simulink model "MCU_vectorControl_dsPIC33AK128MC106_MCLV_48V_300W_2022a"  (R2022a)
settings: Solver=FixedStepDiscrete  StartTime=0.0  StopTime=10.0  FixedStep=50e-6  RelTol=1e-3  EnableMultiTasking=on
undefined symbols (not defined in the file or in its folder): A0, A4, ADC, B0, Bias1, Bias2, C10, C11, C6, C7, C8, control, D11, D12, DiscIntNeverNeededParam, inverter, Max, MaxPer, model, ms, NumBits1, NumBits2, P1, P17, P20, P39, P40, P41, P43, P44, P60, P61, Pin, PosRange1, PosRange2, PWM1_Trg1, Resol, s, Slope1, Slope2, us
libraries: simulink x43, MCHP_Blockset x23
(part 3 of 5)

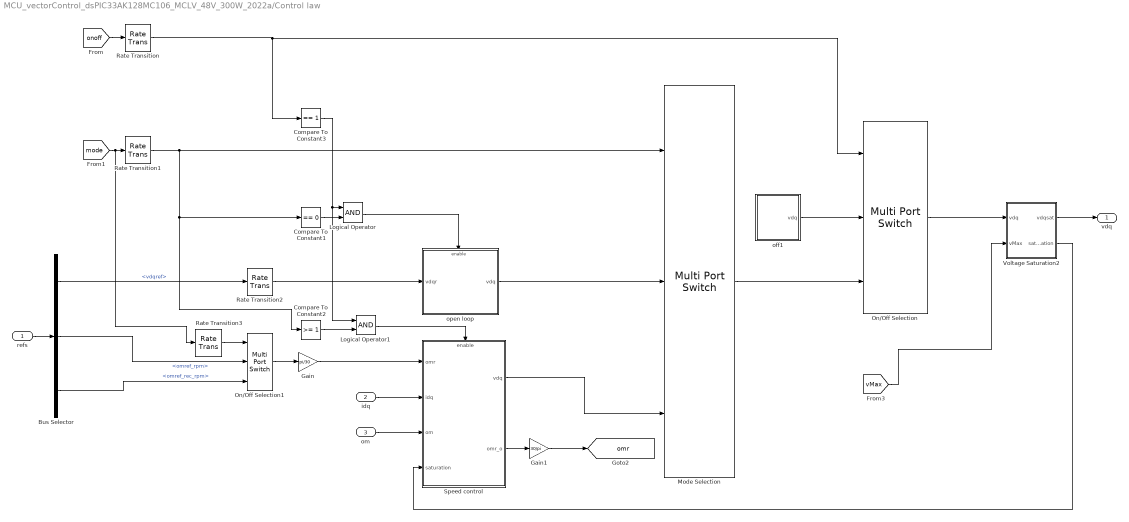
== system MCU_vectorControl_dsPIC33AK128MC106_MCLV_48V_300W_2022a/Control law ==
  refs : Inport
  idq : Inport  Port=2
  om : Inport  Port=3
  Bus Selector : BusSelector  OutputSignals=vdqref,omref.omref_rpm,omref.omref_rec_rpm
  Compare To Constant1 : simulink/Logic and Bit Operations/Compare To Constant  relop===  const=0  OutDataTypeStr=boolean
  Compare To Constant2 : simulink/Logic and Bit Operations/Compare To Constant  relop=>=  const=1  OutDataTypeStr=boolean
  Compare To Constant3 : simulink/Logic and Bit Operations/Compare To Constant  relop===  const=1  OutDataTypeStr=boolean
  Gain : Gain  Gain=pi/30
  Gain1 : Gain  Gain=30/pi
  Logical Operator : Logic  AllPortsSameDT=off  OutDataTypeStr=boolean
  Logical Operator1 : Logic  AllPortsSameDT=off  OutDataTypeStr=boolean
  Mode Selection : MultiPortSwitch  DataPortOrder=Zero-based contiguous  Inputs=2  DiagnosticForDefault=None  zeroidx=on  SaturateOnIntegerOverflow=off  InputSameDT=off
  On/Off Selection : MultiPortSwitch  DataPortOrder=Zero-based contiguous  Inputs=2  DiagnosticForDefault=None  zeroidx=on  SaturateOnIntegerOverflow=off  InputSameDT=off
  On/Off Selection1 : MultiPortSwitch  DataPortOrder=Specify indices  Inputs=2  DataPortIndices={1,2}  DiagnosticForDefault=None  SaturateOnIntegerOverflow=off  InputSameDT=off
  Rate Transition{,1..3} (4 alike) : RateTransition
  Speed control : Subsystem
      settings: PortSchema="{\"entries\":[{\"content\":{\"sides\":[{\"content\":{\"connectorIds\":[\"In1\",\"In2\",\"In3\",\"In4\"]},\"type\":\"ConnectorPlacement.EquallySpacedRectSide\",\"uuid\":\"e7aaa2d5-acdd-4a4d-91b1-423dc6f26e4f\"},{\"content\":{\"connectorIds\":[\"Out1\",\"Out2\"],\"side\":\"RIGHT\"},\"type\":\"ConnectorPlacement.EquallySpacedRectSide\",\"uuid\":\"81691e4d-c138-404c-a913-2433211e99ad\"},{\"content\":{\"connectorIds\":[\"In5\"],\"side\":\"TOP\"},\"type\":\"ConnectorPlacement.EquallySpacedRectSide\",\"uuid\":\"67eaf657-96ad-4741-9677-f3dc17f9f096\"}]},\"type\":\"ConnectorPlacement.EquallySpacedConnector\",\"uuid\":\"09d68ba6-6bd5-4801-b033-56cd43b3cecf\"}],\"packageUris\":[\"http://schema.mathworks.com/mf0/Connector/R2020b\"],\"version\":\"1.0\"}"
  Voltage Saturation2 : Subsystem
  off1 : Subsystem
  open loop : Subsystem
  vdq : Outport  VectorParamsAs1DForOutWhenUnconnected=off
  tag scope: omr=global
  wires:
  On/Off Selection/1 -> Voltage Saturation2/1(vdq)
  [vMax] -> Voltage Saturation2/2(vMax)
  Speed control/1(vdq) -> Mode Selection/3
  Voltage Saturation2/2(saturation) -> Speed control/4(saturation)
  idq/1 -> Speed control/2(idq)
  om/1 -> Speed control/3(om)
  Logical Operator1/1 -> Speed control/5(enable)
  Compare To Constant3/1 -> Logical Operator/1, Logical Operator1/1
  Compare To Constant1/1 -> Logical Operator/2
  Bus Selector/1 -> Rate Transition2/1  "<vdqref>"
  [onoff] -> Rate Transition/1
  open loop/1(vdq) -> Mode Selection/2
  off1/1(vdq) -> On/Off Selection/2
  Mode Selection/1 -> On/Off Selection/3
  Logical Operator/1 -> open loop/Enable
  Compare To Constant2/1 -> Logical Operator1/2
  [mode] -> Rate Transition3/1, Rate Transition1/1
  Voltage Saturation2/1(vdqsat) -> vdq/1
  Rate Transition/1 -> Compare To Constant3/1, On/Off Selection/1
  Rate Transition1/1 -> Mode Selection/1, Compare To Constant2/1, Compare To Constant1/1
  Rate Transition2/1 -> open loop/1(vdqr)
  refs/1 -> Bus Selector/1
  Bus Selector/2 -> On/Off Selection1/2  "<omref_rpm>"
  Bus Selector/3 -> On/Off Selection1/3  "<omref_rec_rpm>"
  On/Off Selection1/1 -> Gain/1
  Gain/1 -> Speed control/1(omr)
  Speed control/2(omr_o) -> Gain1/1
  Gain1/1 -> [omr]
  Rate Transition3/1 -> On/Off Selection1/1

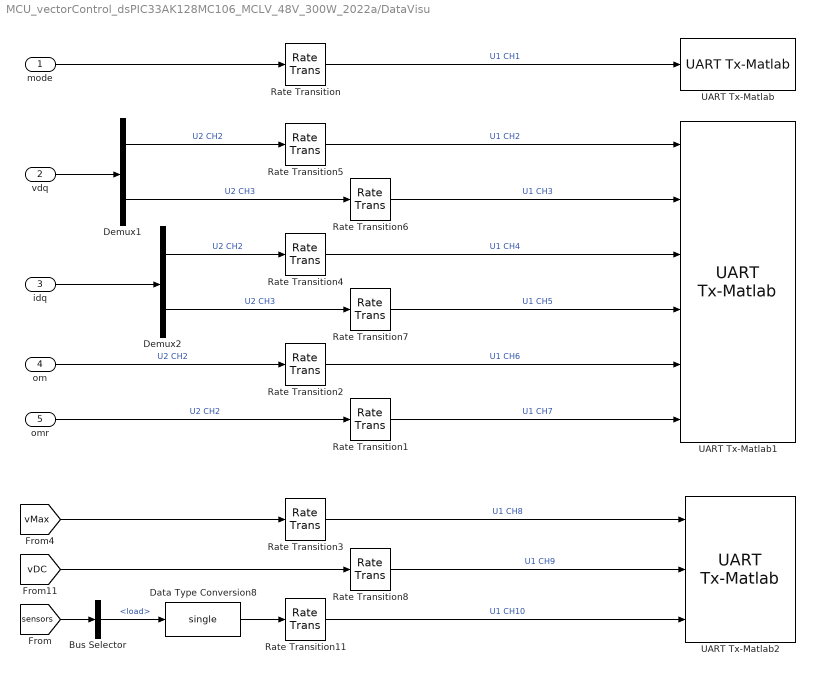
== system MCU_vectorControl_dsPIC33AK128MC106_MCLV_48V_300W_2022a/DataVisu ==
  mode : Inport
  vdq : Inport  Port=2
  idq : Inport  Port=3
  om : Inport  Port=4
  omr : Inport  Port=5
  Bus Selector : BusSelector  OutputSignals=MCU.load
  Data Type Conversion8 : DataTypeConversion  OutDataTypeStr=single  SaturateOnIntegerOverflow=off  RndMeth=Floor
  Demux1 : Demux  Outputs=2
  Demux2 : Demux  Outputs=2
  Rate Transition{,1..8,11} (10 alike) : RateTransition
  UART Tx-Matlab : MCHP_Blockset/BUS UART/UART Tx-Matlab  UART_REF=1  CHANNELS=[1]  AllOrNothing=off  SampleTime=.01  MCHP_MASTERLINK=MCU_vectorControl_dsPIC33AK128MC106_MCLV_48V_300W_2022a/BOARD MCLV-48V-300W dsPIC33AK128MC106 MC DIM/Microchip Master  MCHP_COMPILED_INFO="CompiledSampleTime= [0.010000000000000000208   0 ];CompiledInportDataTypes=[  3 ];CompiledInportDataWidth=[1];"
      settings: SourceProductName=MPLAB Device Blocks for Simulink
  UART Tx-Matlab1 : MCHP_Blockset/BUS UART/UART Tx-Matlab  UART_REF=1  CHANNELS=[2:7]  AllOrNothing=off  SampleTime=0.001  MCHP_MASTERLINK=MCU_vectorControl_dsPIC33AK128MC106_MCLV_48V_300W_2022a/BOARD MCLV-48V-300W dsPIC33AK128MC106 MC DIM/Microchip Master  MCHP_COMPILED_INFO="CompiledSampleTime= [0.0010000000000000000208   0 ];CompiledInportDataTypes=[  1   1   1   1   1   1 ];CompiledInportDataWidth=[1  1  1  1  1  1];"
      settings: SourceProductName=MPLAB Device Blocks for Simulink
  UART Tx-Matlab2 : MCHP_Blockset/BUS UART/UART Tx-Matlab  UART_REF=1  CHANNELS=[8:10]  AllOrNothing=off  SampleTime=.01  MCHP_MASTERLINK=MCU_vectorControl_dsPIC33AK128MC106_MCLV_48V_300W_2022a/BOARD MCLV-48V-300W dsPIC33AK128MC106 MC DIM/Microchip Master  MCHP_COMPILED_INFO="CompiledSampleTime= [0.010000000000000000208   0 ];CompiledInportDataTypes=[  1   1   1 ];CompiledInportDataWidth=[1  1  1];"
      settings: SourceProductName=MPLAB Device Blocks for Simulink
  wires:
  vdq/1 -> Demux1/1
  idq/1 -> Demux2/1
  Demux2/2 -> Rate Transition7/1  "U2 CH3"
  Demux2/1 -> Rate Transition4/1  "U2 CH2"
  Rate Transition5/1 -> UART Tx-Matlab1/1  "U1 CH2"
  Demux1/2 -> Rate Transition6/1  "U2 CH3"
  Rate Transition6/1 -> UART Tx-Matlab1/2  "U1 CH3"
  Rate Transition4/1 -> UART Tx-Matlab1/3  "U1 CH4"
  Demux1/1 -> Rate Transition5/1  "U2 CH2"
  Rate Transition7/1 -> UART Tx-Matlab1/4  "U1 CH5"
  Rate Transition2/1 -> UART Tx-Matlab1/5  "U1 CH6"
  om/1 -> Rate Transition2/1  "U2 CH2"
  Rate Transition/1 -> UART Tx-Matlab/1  "U1 CH1"
  mode/1 -> Rate Transition/1
  omr/1 -> Rate Transition1/1  "U2 CH2"
  Rate Transition1/1 -> UART Tx-Matlab1/6  "U1 CH7"
  [vDC] -> Rate Transition8/1
  [vMax] -> Rate Transition3/1
  Rate Transition3/1 -> UART Tx-Matlab2/1  "U1 CH8"
  Rate Transition8/1 -> UART Tx-Matlab2/2  "U1 CH9"
  Bus Selector/1 -> Data Type Conversion8/1  "<load>"
  Rate Transition11/1 -> UART Tx-Matlab2/3  "U1 CH10"
  [sensors] -> Bus Selector/1
  Data Type Conversion8/1 -> Rate Transition11/1

== system MCU_vectorControl_dsPIC33AK128MC106_MCLV_48V_300W_2022a/Heart-beat 5Hz Blinking ==
  Delay : Delay  DelayLength=1  InitialCondition=0  SampleTime=.1
  Logical Operator : Logic  Operator=NOT  AllPortsSameDT=off  OutDataTypeStr=boolean
  Rate Transition2 : RateTransition  Deterministic=off  OutPortSampleTime=0.01
  LED1 : Outport  VectorParamsAs1DForOutWhenUnconnected=off
  wires:
  Delay/1 -> Logical Operator/1
  Logical Operator/1 -> Delay/1, Rate Transition2/1
  Rate Transition2/1 -> LED1/1

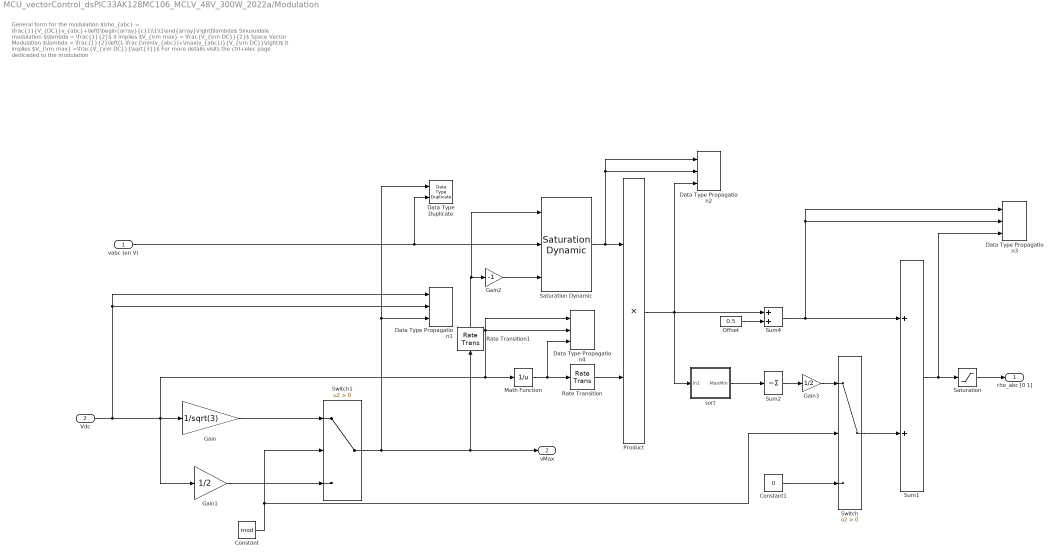
== system MCU_vectorControl_dsPIC33AK128MC106_MCLV_48V_300W_2022a/Modulation ==
  note: General form for the modulation
      | $\rho_{abc} = \frac{1}{V_{DC}}v_{abc}+\left[\begin{array}{c}1\\1\\1\end{array}\right]\lambda$
      | Sinusoidale modulation
      | $\lambda = \frac{1}{2}$ it implies $V_{\rm max} = \frac{V_{\rm DC}}{2}$
      | Space Vector Modulation
      | $\lambda = \frac{1}{2}\left(1-\frac{\min(v_{abc})+\max(v_{abc})}{V_{\rm DC}}\right)$ it implies $V_{\rm max} =\frac{V_{\rm DC}}{\sqrt{3}}$
      | For more details visits the ctrl+elec page dedicaded to the modulation
  "vabc (en V) " : Inport
  Vdc : Inport  Port=2
  Constant : Constant  Value=mod  OutDataTypeStr=boolean
  Constant1 : Constant  Value=0  OutDataTypeStr=Inherit: Inherit via back propagation
  Data Type Duplicate : DataTypeDuplicate
  Data Type Propagation1 : simulink/Signal Attributes/Data Type Propagation  PropDataType=fixdt(1, 16)  IfRefDouble=double  IfRefSingle=single  IsSigned=TRUE  NumBitsBase=max([NumBits1 NumBits2])  NumBitsMult=1  NumBitsAdd=0  NumBitsAllowFinal=[1:128]  PropScaling=2^-(15-ceil(log2(inverter.vDC/sqrt(3))))  ValuesUsedBestPrec=[100 -100]  SlopeBase=max([PosRange1 PosRange2])  SlopeMult=1/sqrt(3)  SlopeAdd=0  BiasBase=Bias1  BiasMult=1  BiasAdd=0
  Data Type Propagation2 : simulink/Signal Attributes/Data Type Propagation  PropDataType=fixdt(1, 16)  IfRefDouble=double  IfRefSingle=single  IsSigned=TRUE  NumBitsBase=max([NumBits1 NumBits2])  NumBitsMult=1  NumBitsAdd=0  NumBitsAllowFinal=[1:128]  PropScalingMode=Specify via dialog  PropScaling=2^-14  ValuesUsedBestPrec=[100 -100]  SlopeBase=Slope1/Slope2  SlopeMult=1  SlopeAdd=0  BiasBase=Bias1  BiasMult=1  BiasAdd=0
  Data Type Propagation3 : simulink/Signal Attributes/Data Type Propagation  PropDataType=fixdt(1, 16)  IfRefDouble=double  IfRefSingle=single  IsSigned=FALSE  NumBitsBase=max([NumBits1 NumBits2])  NumBitsMult=1  NumBitsAdd=0  NumBitsAllowFinal=[1:128]  PropScalingMode=Specify via dialog  PropScaling=2^-14  ValuesUsedBestPrec=[100 -100]  SlopeBase=Slope1/Slope2  SlopeMult=1  SlopeAdd=0  BiasBase=Bias1  BiasMult=1  BiasAdd=0
  Data Type Propagation4 : simulink/Signal Attributes/Data Type Propagation  PropDataType=fixdt(1, 16)  IfRefDouble=double  IfRefSingle=single  IsSigned=FALSE  NumBitsBase=max([NumBits1 NumBits2])  NumBitsMult=1  NumBitsAdd=0  NumBitsAllowFinal=[1:128]  PropScalingMode=Specify via dialog  PropScaling=2^-16  ValuesUsedBestPrec=[100 -100]  SlopeBase=max([PosRange1 PosRange2])  SlopeMult=1/sqrt(3)  SlopeAdd=0  BiasBase=Bias1  BiasMult=1  BiasAdd=0
  Gain : Gain  Gain=1/sqrt(3)  OutDataTypeStr=Inherit: Same as input
  Gain1 : Gain  Gain=1/2  OutDataTypeStr=Inherit: Same as input
  Gain2 : Gain  Gain=-1  ParamDataTypeStr=int16  OutDataTypeStr=Inherit: Inherit via back propagation
  Gain3 : Gain  Gain=1/2  OutDataTypeStr=Inherit: Same as input
  Math Function : Math  Operator=reciprocal  OutputSignalType=real  OutDataTypeStr=Inherit: Inherit via back propagation  SaturateOnIntegerOverflow=off
  "Offset " : Constant  Value=0.5  OutMin=[0]  OutMax=[1]  OutDataTypeStr=Inherit: Inherit via back propagation
  Product : Product  Inputs=**  OutDataTypeStr=Inherit: Inherit via back propagation  SaturateOnIntegerOverflow=on
  Rate Transition : RateTransition
  Rate Transition1 : RateTransition
  Saturation : Saturate  UpperLimit=1  LowerLimit=0
  Saturation Dynamic : simulink/Discontinuities/Saturation Dynamic  OutMin=[]  OutMax=[]  OutDataTypeStr=Inherit: Same as second input  OutDataType=fixdt(1, 16)  OutScaling=2^-10  DoSatur=off
  Sum1 : Sum  OutMin=[0]  OutMax=[1]  OutDataTypeStr=Inherit: Inherit via back propagation  InputSameDT=on  SaturateOnIntegerOverflow=on
  Sum2 : Sum  Inputs=-  OutMin=[-1]  OutMax=[1]  InputSameDT=on  SaturateOnIntegerOverflow=on  OutDataTypeStr=Inherit: Same as first input
  Sum4 : Sum  OutMin=[-1]  OutMax=[1]  InputSameDT=on  SaturateOnIntegerOverflow=on  OutDataTypeStr=Inherit: Same as first input
  Switch : Switch  Criteria=u2 > Threshold  SaturateOnIntegerOverflow=off  InputSameDT=off
  Switch1 : Switch  Criteria=u2 > Threshold  OutDataTypeStr=Inherit: Inherit via back propagation  SaturateOnIntegerOverflow=off  InputSameDT=off
  sort : Subsystem
  rho_abc [0 1] : Outport  VectorParamsAs1DForOutWhenUnconnected=off
  vMax : Outport  Port=2  VectorParamsAs1DForOutWhenUnconnected=off
  wires:
  Sum1/1 -> Saturation/1, Data Type Propagation3/3
  Vdc/1 -> Data Type Propagation1/2, Data Type Propagation1/1, Gain/1, Math Function/1, Data Type Propagation4/2, Data Type Propagation4/1, Gain1/1
  Gain3/1 -> Switch/1
  Saturation/1 -> rho_abc [0 1]/1
  Saturation Dynamic/1 -> Product/1, Data Type Propagation2/1, Data Type Propagation2/2
  Gain1/1 -> Switch1/3
  Gain/1 -> Switch1/1
  sort/1(MaxMin) -> Sum2/1
  Sum2/1 -> Gain3/1
  Sum4/1 -> Data Type Propagation3/2, Data Type Propagation3/1, Sum1/1
  Constant1/1 -> Switch/3
  Switch/1 -> Sum1/2
  "Offset "/1 -> Sum4/2
  Product/1 -> Data Type Propagation2/3, Sum4/1, sort/1(In1)
  Gain2/1 -> Saturation Dynamic/3
  Math Function/1 -> Data Type Propagation4/3, Rate Transition/1
  Switch1/1 -> Rate Transition1/1, vMax/1, Data Type Propagation1/3, Data Type Duplicate/1
  Constant/1 -> Switch1/2, Switch/2
  "vabc (en V) "/1 -> Data Type Duplicate/2, Saturation Dynamic/2
  Rate Transition/1 -> Product/2
  Rate Transition1/1 -> Saturation Dynamic/1, Gain2/1

== system MCU_vectorControl_dsPIC33AK128MC106_MCLV_48V_300W_2022a/Motor Choice + Gain Tunning ==

== system MCU_vectorControl_dsPIC33AK128MC106_MCLV_48V_300W_2022a/Park ==
  xab(c) : Inport
  P(pth) : Inport  Port=2
  Clarke : Subsystem
  Park : Subsystem
  idq : Outport
  wires:
  Park/1(xdq) -> idq/1  "idq"
  P(pth)/1 -> Park/2(P(pth))
  xab(c)/1 -> Clarke/1(xab(c))
  Clarke/1(xalphabeta) -> Park/1(xalphabeta)

== system MCU_vectorControl_dsPIC33AK128MC106_MCLV_48V_300W_2022a/Park inverse ==
  xdq : Inport
  P(pth) : Inport  Port=2
  Clarke Inverse : Subsystem
  Park inverse : Subsystem
  xabc : Outport
  wires:
  Park inverse/1(xalpahbeta) -> Clarke Inverse/1(xalphabeta)
  xdq/1 -> Park inverse/1(xdq)
  Clarke Inverse/1(xabc) -> xabc/1
  P(pth)/1 -> Park inverse/2(P(pth))

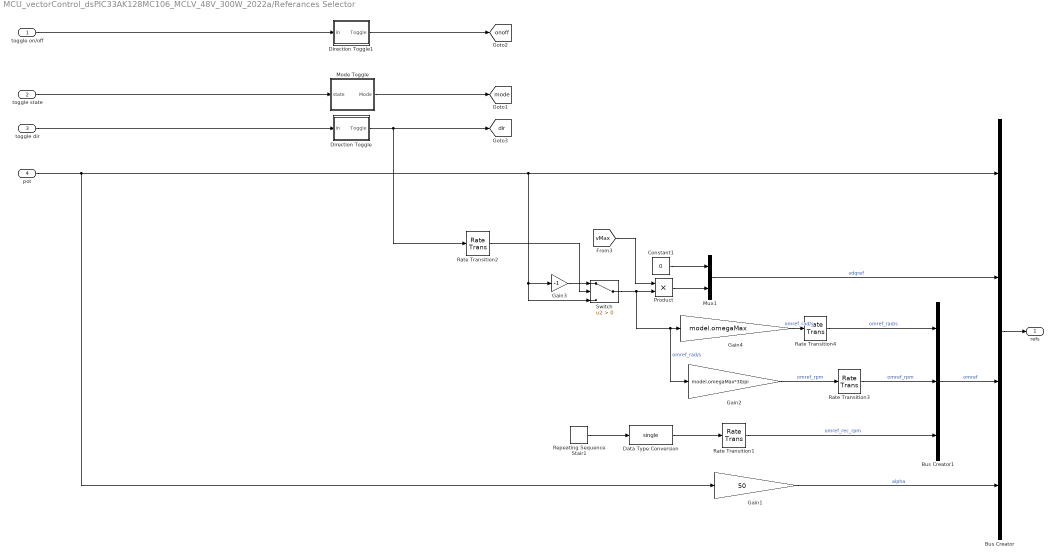
== system MCU_vectorControl_dsPIC33AK128MC106_MCLV_48V_300W_2022a/Referances Selector ==
  toggle on/off : Inport  SampleTime=.01
  toggle state : Inport  Port=2  SampleTime=.01
  toggle dir : Inport  Port=3  SampleTime=.01
  pot : Inport  Port=4
  Bus Creator : BusCreator  Inputs=4
  Bus Creator1 : BusCreator  Inputs=3
  Constant1 : Constant  Value=0  OutDataTypeStr=Inherit: Inherit via back propagation
  Data Type Conversion : DataTypeConversion  OutDataTypeStr=single  SaturateOnIntegerOverflow=off  RndMeth=Floor
  Direction Toggle : Subsystem
  Direction Toggle1 : Subsystem
  Gain1 : Gain  Gain=50
  Gain2 : Gain  Gain=model.omegaMax*30/pi
  Gain3 : Gain  Gain=-1  OutDataTypeStr=Inherit: Inherit via back propagation  SaturateOnIntegerOverflow=on
  Gain4 : Gain  Gain=model.omegaMax
  Mode Toggle : Subsystem
  Mux1 : Mux  Inputs=2
  Product : Product  OutDataTypeStr=Inherit: Same as first input
  Rate Transition1 : RateTransition  Deterministic=off  OutPortSampleTime=0.001
  Rate Transition2 : RateTransition  Integrity=off  OutPortSampleTime=0.001
  Rate Transition3 : RateTransition  OutPortSampleTime=0.001
  Rate Transition4 : RateTransition  OutPortSampleTime=0.001
  Repeating Sequence Stair1 : simulink/Sources/Repeating Sequence Stair  OutValues=[1000 4000].'  tsamp=2  OutMin=[]  OutMax=[]  OutDataTypeStr=single  OutputDataTypeScalingMode=single  OutDataType=fixdt(0,8)  ConRadixGroup=Best Precision: Vector-wise  OutScaling=2^-12
  Switch : Switch  Criteria=u2 > Threshold  OutDataTypeStr=Inherit: Inherit via back propagation  SaturateOnIntegerOverflow=off  InputSameDT=off
  refs : Outport
  tag scope: dir=global, mode=global, onoff=global
  wires:
  toggle dir/1 -> Direction Toggle/1(in)
  toggle state/1 -> Mode Toggle/1(state)
  toggle on/off/1 -> Direction Toggle1/1(in)
  Rate Transition2/1 -> Switch/2
  [vMax] -> Product/1
  Gain3/1 -> Switch/1
  Mode Toggle/1(Mode) -> [mode]
  Direction Toggle1/1(Toggle) -> [onoff]
  Constant1/1 -> Mux1/1
  Mux1/1 -> Bus Creator/2  "vdqref"
  Direction Toggle/1(Toggle) -> [dir], Rate Transition2/1
  Switch/1 -> Gain2/1, Gain4/1, Product/2  "omref_rad/s"
  pot/1 -> Gain1/1, Switch/3, Gain3/1, Bus Creator/1
  Bus Creator/1 -> refs/1
  Bus Creator1/1 -> Bus Creator/3  "omref"
  Gain2/1 -> Rate Transition3/1  "omref_rpm"
  Gain4/1 -> Rate Transition4/1  "omref_rad/s"
  Product/1 -> Mux1/2
  Gain1/1 -> Bus Creator/4  "alpha"
  Repeating Sequence Stair1/1 -> Data Type Conversion/1
  Rate Transition1/1 -> Bus Creator1/3  "omref_rec_rpm"
  Data Type Conversion/1 -> Rate Transition1/1
  Rate Transition3/1 -> Bus Creator1/2  "omref_rpm"
  Rate Transition4/1 -> Bus Creator1/1  "omref_rad/s"

== system MCU_vectorControl_dsPIC33AK128MC106_MCLV_48V_300W_2022a/Rot ==
  sin cos : Inport
  Demux3 : Demux  Outputs=2
  Gain : Gain  Gain=-1  OutDataTypeStr=Inherit: Same as input
  Mux1 : Mux
  Reshape : Reshape  OutputDimensionality=Customize  OutputDimensions=[2,2]
  "cos sin -sin cos " : Outport  PortDimensions=[2 2]
  wires:
  Reshape/1 -> "cos sin -sin cos "/1
  sin cos/1 -> Demux3/1
  Gain/1 -> Mux1/2
  Mux1/1 -> Reshape/1
  Demux3/1 -> Mux1/3, Gain/1
  Demux3/2 -> Mux1/4, Mux1/1
